simulink model "simulink_validacao"  (R2016a)
settings: Solver=VariableStepAuto  StartTime=0.0  StopTime=10.0  RelTol=1e-3
values from neighbouring files (symbols this model uses):
  f_mol_ar = [0.79 0.21 0.0 0 0 0 0 0]    [codigo_validacao.m]
  f_mol_gas = [0.76 0 0 0 0.11 0.13 0 0]    [codigo_validacao.m]
  m_c = 0.3    [codigo_validacao.m]
  m_f = 0.01    [codigo_validacao.m]
  N = 0.82    [codigo_validacao.m]
  Pc_i = 368000    [codigo_validacao.m]
  Ph_i = 105000    [codigo_validacao.m]
  Tc_i = 358.15    [codigo_validacao.m]
  Th_i = 584.817    [codigo_validacao.m]
(part 1 of 4)
settings Model: Creator=Janderson Honório  LastModifiedBy=Janderson Honório

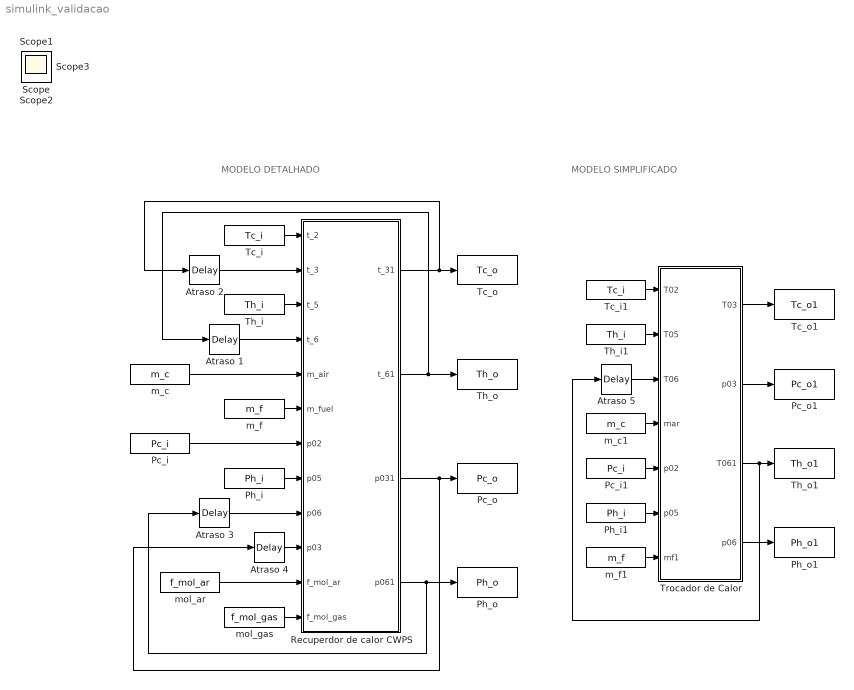
== system simulink_validacao ==
  note: MODELO DETALHADO
  note: MODELO SIMPLIFICADO
  Atraso 1 : TransportDelay  DelayTime=0.1  InitialOutput=400  TransDelayFeedthrough=on
  Atraso 2 : TransportDelay  DelayTime=0.1  InitialOutput=650  TransDelayFeedthrough=on
  Atraso 3 : TransportDelay  DelayTime=0.1  InitialOutput=300000  TransDelayFeedthrough=on
  Atraso 4 : TransportDelay  DelayTime=0.1  InitialOutput=100000  TransDelayFeedthrough=on
  Atraso 5 : TransportDelay  DelayTime=0.1  InitialOutput=500  TransDelayFeedthrough=on
  Pc_i : Constant  Value=Pc_i
  Pc_i1 : Constant  Value=Pc_i
  Pc_o : ToWorkspace  VariableName=Pc_o  SampleTime=-1
      settings: Save2DSignal=2-D array (concatenate along first dimension)
  Pc_o1 : ToWorkspace  VariableName=Pc_o1  SampleTime=-1
      settings: Save2DSignal=2-D array (concatenate along first dimension)
  Ph_i : Constant  Value=Ph_i
  Ph_i1 : Constant  Value=Ph_i
  Ph_o : ToWorkspace  VariableName=Ph_o  SampleTime=-1
      settings: Save2DSignal=2-D array (concatenate along first dimension)
  Ph_o1 : ToWorkspace  VariableName=Ph_o1  SampleTime=-1
      settings: Save2DSignal=2-D array (concatenate along first dimension)
  Recuperdor de calor CWPS : Subsystem
  Tc_i : Constant  Value=Tc_i
  Tc_i1 : Constant  Value=Tc_i
  Tc_o : ToWorkspace  VariableName=Tc_o  SampleTime=-1
      settings: Save2DSignal=2-D array (concatenate along first dimension)
  Tc_o1 : ToWorkspace  VariableName=Tc_o1  SampleTime=-1
      settings: Save2DSignal=2-D array (concatenate along first dimension)
  Th_i : Constant  Value=Th_i
  Th_i1 : Constant  Value=Th_i
  Th_o : ToWorkspace  VariableName=Th_o  SampleTime=-1
      settings: Save2DSignal=2-D array (concatenate along first dimension)
  Th_o1 : ToWorkspace  VariableName=Th_o1  SampleTime=-1
      settings: Save2DSignal=2-D array (concatenate along first dimension)
  Trocador de Calor : Subsystem
  m_c : Constant  Value=m_c
  m_c1 : Constant  Value=m_c
  m_f : Constant  Value=m_f
  m_f1 : Constant  Value=m_f
  mol_ar : Constant  Value=f_mol_ar
  mol_gas : Constant  Value=f_mol_gas
  Scope{,1..3} (4 alike) : Scope
  wires:
  Recuperdor de calor CWPS/1(t_31) -> Tc_o/1, Atraso 2/1
  Recuperdor de calor CWPS/2(t_61) -> Th_o/1, Atraso 1/1
  Recuperdor de calor CWPS/4(p061) -> Ph_o/1, Atraso 3/1
  Atraso 2/1 -> Recuperdor de calor CWPS/2(t_3)
  Th_i/1 -> Recuperdor de calor CWPS/3(t_5)
  Atraso 1/1 -> Recuperdor de calor CWPS/4(t_6)
  Atraso 4/1 -> Recuperdor de calor CWPS/10(p03)
  Atraso 3/1 -> Recuperdor de calor CWPS/9("p06 ")
  mol_ar/1 -> Recuperdor de calor CWPS/11(f_mol_ar)
  mol_gas/1 -> Recuperdor de calor CWPS/12(f_mol_gas)
  Tc_i/1 -> Recuperdor de calor CWPS/1(t_2)
  m_f/1 -> Recuperdor de calor CWPS/6(m_fuel)
  m_c/1 -> Recuperdor de calor CWPS/5("m_air ")
  Ph_i/1 -> Recuperdor de calor CWPS/8(p05)
  Pc_i/1 -> Recuperdor de calor CWPS/7(p02)
  Trocador de Calor/3(T061) -> Atraso 5/1, Th_o1/1
  Atraso 5/1 -> Trocador de Calor/3(T06)
  Tc_i1/1 -> Trocador de Calor/1(T02)
  Th_i1/1 -> Trocador de Calor/2(T05)
  m_c1/1 -> Trocador de Calor/4(mar)
  m_f1/1 -> Trocador de Calor/7(mf1)
  Pc_i1/1 -> Trocador de Calor/5(p02)
  Ph_i1/1 -> Trocador de Calor/6(p05)
  Trocador de Calor/1(T03) -> Tc_o1/1
  Trocador de Calor/2(p03) -> Pc_o1/1
  Trocador de Calor/4(p06) -> Ph_o1/1
  Recuperdor de calor CWPS/3(p031) -> Pc_o/1, Atraso 4/1

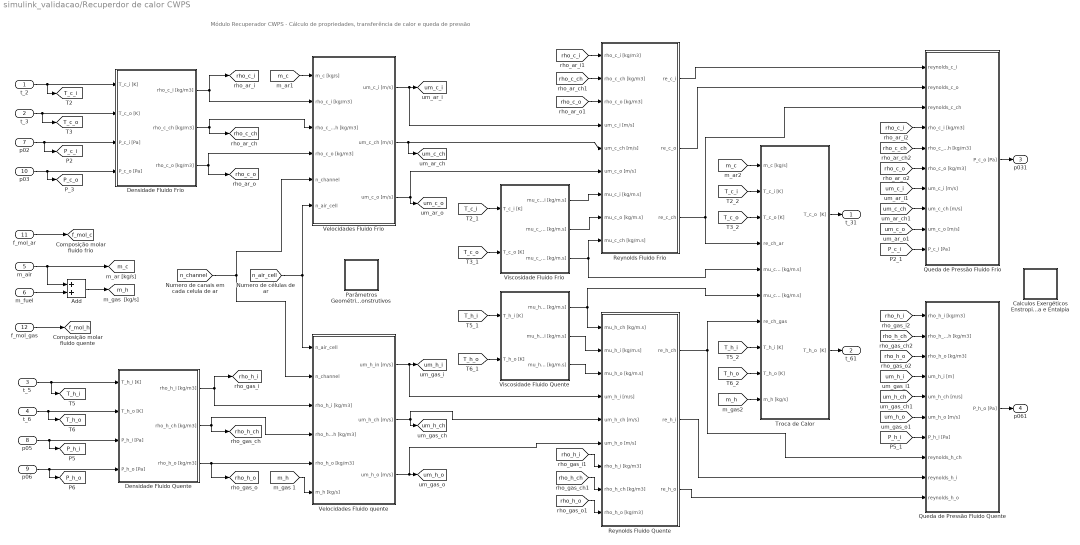
== system simulink_validacao/Recuperdor de calor CWPS ==
  note: Módulo Recuperador CWPS - Cálculo de propriedades, transferência de calor e queda de pressão
  t_2 : Inport
  t_3 : Inport  Port=2
  t_5 : Inport  Port=3
  t_6 : Inport  Port=4
  "m_air " : Inport  Port=5
  m_fuel : Inport  Port=6
  p02 : Inport  Port=7
  p05 : Inport  Port=8
  "p06 " : Inport  Port=9
  p03 : Inport  Port=10
  f_mol_ar : Inport  Port=11
  f_mol_gas : Inport  Port=12
  Add : Sum
  Calculos Exergéticos Enstropia e Entalpia : Subsystem
  Densidade Fluido Frio : Subsystem
  Densidade Fluido Quente : Subsystem
  Parâmetros Geométricos e Construtivos : Subsystem
  Queda de Pressão Fluido Frio : Subsystem
  Queda de Pressão Fluido Quente : Subsystem
  Reynolds Fluido Frio : Subsystem
  Reynolds Fluido Quente : Subsystem
  Troca de Calor : Subsystem
  Velocidades Fluido Frio : Subsystem
  Velocidades Fluido quente : Subsystem
  "Viscosidade Fluido Frio " : Subsystem
  Viscosidade Fluido Quente : Subsystem
  t_31 : Outport
  t_61 : Outport  Port=2
  p031 : Outport  Port=3
  p061 : Outport  Port=4
  tag scope: P_c_i=global, P_c_o=global, P_h_i=global, P_h_o=global, T_c_i=global, T_c_o=global, T_h_i=global, T_h_o=global, f_mol_c=global, f_mol_h=global, m_c=global, m_h=global, rho_c_ch=global, rho_c_i=global, rho_c_o=global, rho_h_ch=global, rho_h_i=global, rho_h_o=global, um_c_ch=global, um_c_i=global, um_c_o=global, um_h_ch=global, um_h_i=global, um_h_o=global
  wires:
  t_3/1 -> [T_c_o], Densidade Fluido Frio/2(T_c_o [K])
  t_2/1 -> Densidade Fluido Frio/1(T_c_i [K]), [T_c_i]
  p02/1 -> [P_c_i], Densidade Fluido Frio/3(P_c_i [Pa])
  t_6/1 -> [T_h_o], Densidade Fluido Quente/2(T_h_o [K])
  t_5/1 -> [T_h_i], Densidade Fluido Quente/1(T_h_i [K])
  "p06 "/1 -> [P_h_o], Densidade Fluido Quente/4(P_h_o [Pa])
  Densidade Fluido Frio/2(rho_c_ch [kg/m3]) -> Velocidades Fluido Frio/3(rho_c_ch [kg/m3]), [rho_c_ch]
  Densidade Fluido Frio/3(rho_c_o [kg/m3]) -> [rho_c_o], Velocidades Fluido Frio/4("rho_c_o [kg/m3] ")
  Densidade Fluido Quente/2(rho_h_ch [kg/m3]) -> Velocidades Fluido quente/4(rho_h_ch [kg/m3]), [rho_h_ch]
  Densidade Fluido Quente/3(rho_h_o [kg/m3]) -> Velocidades Fluido quente/5(rho_h_o [kg/m3]), [rho_h_o]
  Densidade Fluido Quente/1(rho_h_i [kg/m3]) -> [rho_h_i], Velocidades Fluido quente/3(rho_h_i [kg/m3])
  [n_air_cell] -> Velocidades Fluido quente/1(n_air_cell), Velocidades Fluido Frio/6(n_air_cell)
  [n_channel] -> Velocidades Fluido quente/2(n_channel), Velocidades Fluido Frio/5(n_channel)
  Velocidades Fluido Frio/1(um_c_i [m/s]) -> [um_c_i], Reynolds Fluido Frio/4(um_c_i [m/s])
  Velocidades Fluido Frio/2(um_c_ch [m/s]) -> [um_c_ch], Reynolds Fluido Frio/5(um_c_ch [m/s])
  Velocidades Fluido Frio/3(um_c_o [m/s]) -> Reynolds Fluido Frio/6(um_c_o [m/s]), [um_c_o]
  Velocidades Fluido quente/1(um_h_in [m/s]) -> [um_h_i], Reynolds Fluido Quente/4(um_h_i [m/s])
  Velocidades Fluido quente/2(um_h_ch [m/s]) -> Reynolds Fluido Quente/5(um_h_ch [m/s]), [um_h_ch]
  Velocidades Fluido quente/3(um_h_o [m/s]) -> Reynolds Fluido Quente/6(um_h_o [m/s]), [um_h_o]
  Queda de Pressão Fluido Quente/1(P_h_o [Pa]) -> p061/1
  p05/1 -> [P_h_i], Densidade Fluido Quente/3(P_h_i [Pa])
  [rho_c_i] -> Reynolds Fluido Frio/1(rho_c_i [kg/m3])
  [rho_c_ch] -> Reynolds Fluido Frio/2(rho_c_ch [kg/m3])
  [rho_c_o] -> Reynolds Fluido Frio/3(rho_c_o [kg/m3])
  [rho_c_i] -> Queda de Pressão Fluido Frio/4(rho_c_i [kg/m3])
  [rho_c_o] -> Queda de Pressão Fluido Frio/6("rho_c_o [kg/m3] ")
  [rho_c_ch] -> Queda de Pressão Fluido Frio/5("rho_c_ch [kg/m3] ")
  [rho_h_i] -> Reynolds Fluido Quente/7(rho_h_i [kg/m3])
  [rho_h_ch] -> Reynolds Fluido Quente/8(rho_h_ch [kg/m3])
  [rho_h_o] -> Reynolds Fluido Quente/9(rho_h_o [kg/m3])
  [rho_h_o] -> Queda de Pressão Fluido Quente/3("rho_h_o [kg/m3] ")
  [rho_h_i] -> Queda de Pressão Fluido Quente/1(rho_h_i [kg/m3])
  [rho_h_ch] -> Queda de Pressão Fluido Quente/2("rho_h_ch [kg/m3] ")
  Troca de Calor/2(T_h_o  [K]) -> t_61/1
  [um_c_i] -> Queda de Pressão Fluido Frio/7(um_c_i [m/s])
  [um_c_ch] -> Queda de Pressão Fluido Frio/8(um_c_ch [m/s])
  [um_c_o] -> Queda de Pressão Fluido Frio/9(um_c_o [m/s])
  [um_h_i] -> Queda de Pressão Fluido Quente/4(um_h_i [m])
  [um_h_ch] -> Queda de Pressão Fluido Quente/5(um_h_ch [m/s])
  [um_h_o] -> Queda de Pressão Fluido Quente/6(um_h_o [m/s])
  [T_c_i] -> "Viscosidade Fluido Frio "/1(T_c_i [K])
  [T_c_o] -> "Viscosidade Fluido Frio "/2(T_c_o [K])
  [P_h_i] -> Queda de Pressão Fluido Quente/7(P_h_i [Pa])
  [P_c_i] -> Queda de Pressão Fluido Frio/10(P_c_i [Pa])
  "m_air "/1 -> Add/1, [m_c]
  [m_c] -> Velocidades Fluido Frio/1(m_c [kg/s])
  [m_h] -> Velocidades Fluido quente/6(m_h [kg/s])
  [m_h] -> Troca de Calor/10(m_h [kg/s])
  Troca de Calor/1(T_c_o  [K]) -> t_31/1
  [m_c] -> Troca de Calor/1(m_c [kg/s])
  [T_h_i] -> Troca de Calor/8(T_h_i [K])
  [T_h_o] -> Troca de Calor/9(T_h_o [K])
  [T_c_i] -> Troca de Calor/2("T_c_i [K] ")
  [T_c_o] -> Troca de Calor/3(T_c_o [K])
  [T_h_i] -> Viscosidade Fluido Quente/1(T_h_i [K])
  [T_h_o] -> Viscosidade Fluido Quente/2(T_h_o [K])
  "Viscosidade Fluido Frio "/2(mu_c_o [kg/m.s]) -> Reynolds Fluido Frio/8(mu_c_o [kg/m.s])
  "Viscosidade Fluido Frio "/3(mu_c_ch [kg/m.s]) -> Troca de Calor/5(mu_ch_c [kg/m.s]), Reynolds Fluido Frio/9(mu_c_ch [kg/m.s])
  "Viscosidade Fluido Frio "/1(mu_c_i [kg/m.s]) -> Reynolds Fluido Frio/7(mu_c_i [kg/m.s])
  Viscosidade Fluido Quente/1(mu_h_ch [kg/m.s]) -> Troca de Calor/6(mu_ch_h [kg/m.s]), Reynolds Fluido Quente/1(mu_h_ch [kg/m.s])
  Viscosidade Fluido Quente/2(mu_h_i [kg/m.s]) -> Reynolds Fluido Quente/2("mu_h_i [kg/m.s] ")
  Viscosidade Fluido Quente/3(mu_h_o [kg/m.s]) -> Reynolds Fluido Quente/3(mu_h_o [kg/m.s])
  Reynolds Fluido Frio/3(re_c_ch) -> Troca de Calor/4(re_ch_ar), Queda de Pressão Fluido Frio/3(reynolds_c_ch)
  Reynolds Fluido Quente/1(re_h_ch) -> Troca de Calor/7(re_ch_gas), Queda de Pressão Fluido Quente/8(reynolds_h_ch)
  Reynolds Fluido Frio/1(re_c_i) -> Queda de Pressão Fluido Frio/1(reynolds_c_i)
  Reynolds Fluido Frio/2(re_c_o) -> Queda de Pressão Fluido Frio/2(reynolds_c_o)
  Reynolds Fluido Quente/2(re_h_i) -> Queda de Pressão Fluido Quente/9(reynolds_h_i)
  Reynolds Fluido Quente/3(re_h_o) -> Queda de Pressão Fluido Quente/10(reynolds_h_o)
  p03/1 -> [P_c_o], Densidade Fluido Frio/4(P_c_o [Pa])
  Densidade Fluido Frio/1(rho_c_i [kg/m3]) -> Velocidades Fluido Frio/2(rho_c_i [kg/m3]), [rho_c_i]
  f_mol_ar/1 -> [f_mol_c]
  f_mol_gas/1 -> [f_mol_h]
  Queda de Pressão Fluido Frio/1(P_c_o [Pa]) -> p031/1
  m_fuel/1 -> Add/2
  Add/1 -> [m_h]

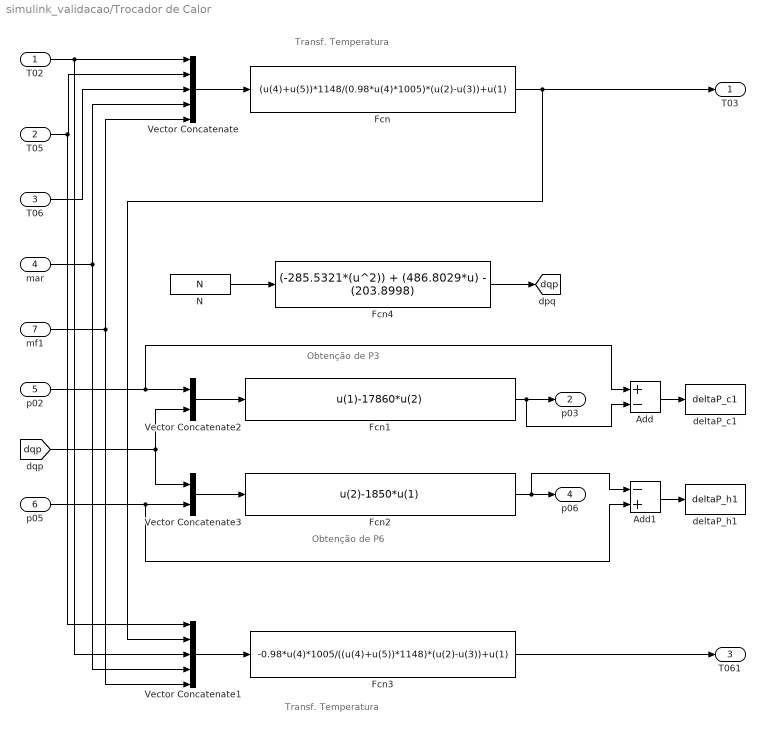
== system simulink_validacao/Trocador de Calor ==
  note: Transf. Temperatura
  note: Obtenção de P3
  note: Obtenção de P6
  note: Transf. Temperatura
  T02 : Inport
  T05 : Inport  Port=2
  T06 : Inport  Port=3
  mar : Inport  Port=4
  p02 : Inport  Port=5
  p05 : Inport  Port=6
  mf1 : Inport  Port=7
  Add : Sum  Inputs=+-
  Add1 : Sum  Inputs=-+
  Fcn : Fcn  Expr=(u(4)+u(5))*1148/(0.98*u(4)*1005)*(u(2)-u(3))+u(1)
  Fcn1 : Fcn  Expr=u(1)-17860*u(2)
  Fcn2 : Fcn  Expr=u(2)-1850*u(1)
  Fcn3 : Fcn  Expr=-0.98*u(4)*1005/((u(4)+u(5))*1148)*(u(2)-u(3))+u(1)
  Fcn4 : Fcn  Expr=(-285.5321*(u^2)) + (486.8029*u) - (203.8998)
  N : Constant  Value=N
  Vector Concatenate : Concatenate  NumInputs=5
  Vector Concatenate1 : Concatenate  NumInputs=5
  Vector Concatenate2 : Concatenate
  Vector Concatenate3 : Concatenate
  deltaP_c1 : ToWorkspace  VariableName=deltaP_c1  SampleTime=-1
      settings: Save2DSignal=2-D array (concatenate along first dimension)
  deltaP_h1 : ToWorkspace  VariableName=deltaP_h1  SampleTime=-1
      settings: Save2DSignal=2-D array (concatenate along first dimension)
  T03 : Outport
  p03 : Outport  Port=2
  T061 : Outport  Port=3
  p06 : Outport  Port=4
  tag scope: dqp=global
  wires:
  Fcn3/1 -> T061/1
  Vector Concatenate/1 -> Fcn/1
  Fcn1/1 -> Add/2, p03/1
  T06/1 -> Vector Concatenate/3
  Fcn2/1 -> Add1/1, p06/1
  Vector Concatenate1/1 -> Fcn3/1
  T05/1 -> Vector Concatenate1/1, Vector Concatenate/2
  Fcn/1 -> Vector Concatenate1/2, T03/1
  T02/1 -> Vector Concatenate1/3, Vector Concatenate/1
  mar/1 -> Vector Concatenate1/4, Vector Concatenate/4
  mf1/1 -> Vector Concatenate1/5, Vector Concatenate/5
  p02/1 -> Add/1, Vector Concatenate2/1
  [dqp] -> Vector Concatenate3/1, Vector Concatenate2/2
  Vector Concatenate2/1 -> Fcn1/1
  p05/1 -> Add1/2, Vector Concatenate3/2
  Vector Concatenate3/1 -> Fcn2/1
  N/1 -> Fcn4/1
  Fcn4/1 -> [dqp]
  Add1/1 -> deltaP_h1/1
  Add/1 -> deltaP_c1/1

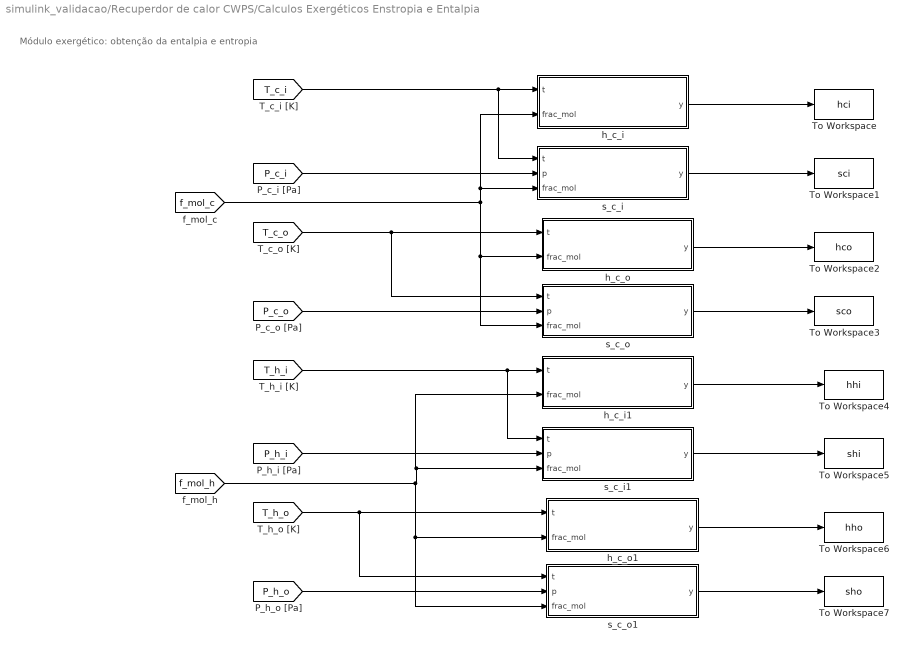
== system simulink_validacao/Recuperdor de calor CWPS/Calculos Exergéticos Enstropia e Entalpia ==
  note: Módulo exergético: obtenção da entalpia e entropia
  To Workspace : ToWorkspace  VariableName=hci  SampleTime=-1
      settings: Save2DSignal=2-D array (concatenate along first dimension)
  To Workspace1 : ToWorkspace  VariableName=sci  SampleTime=-1
      settings: Save2DSignal=2-D array (concatenate along first dimension)
  To Workspace2 : ToWorkspace  VariableName=hco  SampleTime=-1
      settings: Save2DSignal=2-D array (concatenate along first dimension)
  To Workspace3 : ToWorkspace  VariableName=sco  SampleTime=-1
      settings: Save2DSignal=2-D array (concatenate along first dimension)
  To Workspace4 : ToWorkspace  VariableName=hhi  SampleTime=-1
      settings: Save2DSignal=2-D array (concatenate along first dimension)
  To Workspace5 : ToWorkspace  VariableName=shi  SampleTime=-1
      settings: Save2DSignal=2-D array (concatenate along first dimension)
  To Workspace6 : ToWorkspace  VariableName=hho  SampleTime=-1
      settings: Save2DSignal=2-D array (concatenate along first dimension)
  To Workspace7 : ToWorkspace  VariableName=sho  SampleTime=-1
      settings: Save2DSignal=2-D array (concatenate along first dimension)
  h_c_i : MATLAB Function  TreatAsAtomicUnit=on
  h_c_i1 : MATLAB Function  TreatAsAtomicUnit=on
  h_c_o : MATLAB Function  TreatAsAtomicUnit=on
  h_c_o1 : MATLAB Function  TreatAsAtomicUnit=on
  s_c_i : MATLAB Function  TreatAsAtomicUnit=on
  s_c_i1 : MATLAB Function  TreatAsAtomicUnit=on
  s_c_o : MATLAB Function  TreatAsAtomicUnit=on
  s_c_o1 : MATLAB Function  TreatAsAtomicUnit=on
  wires:
  [T_c_i] -> s_c_i/1(t), h_c_i/1(t)
  [f_mol_c] -> s_c_o/3(frac_mol), h_c_o/2(frac_mol), h_c_i/2(frac_mol), s_c_i/3(frac_mol)
  h_c_i/1(y) -> To Workspace/1
  s_c_i/1(y) -> To Workspace1/1
  [P_c_i] -> s_c_i/2(p)
  h_c_o/1(y) -> To Workspace2/1
  s_c_o/1(y) -> To Workspace3/1
  h_c_i1/1(y) -> To Workspace4/1
  s_c_i1/1(y) -> To Workspace5/1
  h_c_o1/1(y) -> To Workspace6/1
  s_c_o1/1(y) -> To Workspace7/1
  [T_c_o] -> h_c_o/1(t), s_c_o/1(t)
  [P_c_o] -> s_c_o/2(p)
  [T_h_i] -> s_c_i1/1(t), h_c_i1/1(t)
  [P_h_i] -> s_c_i1/2(p)
  [f_mol_h] -> s_c_o1/3(frac_mol), h_c_o1/2(frac_mol), s_c_i1/3(frac_mol), h_c_i1/2(frac_mol)
  [T_h_o] -> s_c_o1/1(t), h_c_o1/1(t)
  [P_h_o] -> s_c_o1/2(p)

== system simulink_validacao/Recuperdor de calor CWPS/Densidade Fluido Frio ==
  note: Módulo cálculo de densidades no recuperador - Fluido frio
  T_c_i [K] : Inport
  T_c_o [K] : Inport  Port=2
  P_c_i [Pa] : Inport  Port=3
  P_c_o [Pa] : Inport  Port=4
  Mux : Mux  Inputs=2
  Mux2 : Mux  Inputs=2
  P media fluido frio : Fcn  Expr=(u(1)+u(2))/2
  T media fluido frio : Fcn  Expr=(u(1)+u(2))/2
  densidade_c_ch : MATLAB Function  TreatAsAtomicUnit=on
  densidade_c_i : MATLAB Function  TreatAsAtomicUnit=on
  densidade_c_o : MATLAB Function  TreatAsAtomicUnit=on
  rho_c_i [kg/m3] : Outport
  rho_c_ch [kg/m3] : Outport  Port=2
  rho_c_o [kg/m3] : Outport  Port=3
  wires:
  Mux/1 -> T media fluido frio/1
  T_c_i [K]/1 -> densidade_c_i/1(t), Mux/1
  densidade_c_ch/1(y) -> rho_c_ch [kg/m3]/1
  densidade_c_i/1(y) -> rho_c_i [kg/m3]/1
  densidade_c_o/1(y) -> rho_c_o [kg/m3]/1
  Mux2/1 -> P media fluido frio/1
  T media fluido frio/1 -> densidade_c_ch/1(t)
  P media fluido frio/1 -> densidade_c_ch/2(p)
  T_c_o [K]/1 -> densidade_c_o/1(t), Mux/2
  P_c_i [Pa]/1 -> Mux2/1, densidade_c_i/2(p)
  P_c_o [Pa]/1 -> densidade_c_o/2(p), Mux2/2
  [f_mol_c] -> densidade_c_o/3(frac_mol), densidade_c_ch/3(frac_mol), densidade_c_i/3(frac_mol)

== system simulink_validacao/Recuperdor de calor CWPS/Densidade Fluido Quente ==
  note: Módulo cálculo de densidades no recuperador - Fluido quente
  T_h_i [K] : Inport
  T_h_o [K] : Inport  Port=2
  P_h_i [Pa] : Inport  Port=3
  P_h_o [Pa] : Inport  Port=4
  Mux1 : Mux  Inputs=2
  Mux3 : Mux  Inputs=2
  P media fluido quente : Fcn  Expr=(u(1)+u(2))/2
  T media fluido quente : Fcn  Expr=(u(1)+u(2))/2
  densidade_h_ch : MATLAB Function  TreatAsAtomicUnit=on
  densidade_h_i : MATLAB Function  TreatAsAtomicUnit=on
  densidade_h_o : MATLAB Function  TreatAsAtomicUnit=on
  rho_h_i [kg/m3] : Outport
  rho_h_ch [kg/m3] : Outport  Port=2
  rho_h_o [kg/m3] : Outport  Port=3
  wires:
  Mux1/1 -> T media fluido quente/1
  T_h_i [K]/1 -> Mux1/1, densidade_h_i/1(t)
  Mux3/1 -> P media fluido quente/1
  T media fluido quente/1 -> densidade_h_ch/1(t)
  P media fluido quente/1 -> densidade_h_ch/2(p)
  T_h_o [K]/1 -> densidade_h_o/1(t), Mux1/2
  P_h_i [Pa]/1 -> densidade_h_i/2(p), Mux3/1
  P_h_o [Pa]/1 -> densidade_h_o/2(p), Mux3/2
  densidade_h_i/1(y) -> rho_h_i [kg/m3]/1
  densidade_h_ch/1(y) -> rho_h_ch [kg/m3]/1
  densidade_h_o/1(y) -> rho_h_o [kg/m3]/1
  [f_mol_h] -> densidade_h_i/3(frac_mol), densidade_h_o/3(frac_mol), densidade_h_ch/3(frac_mol)

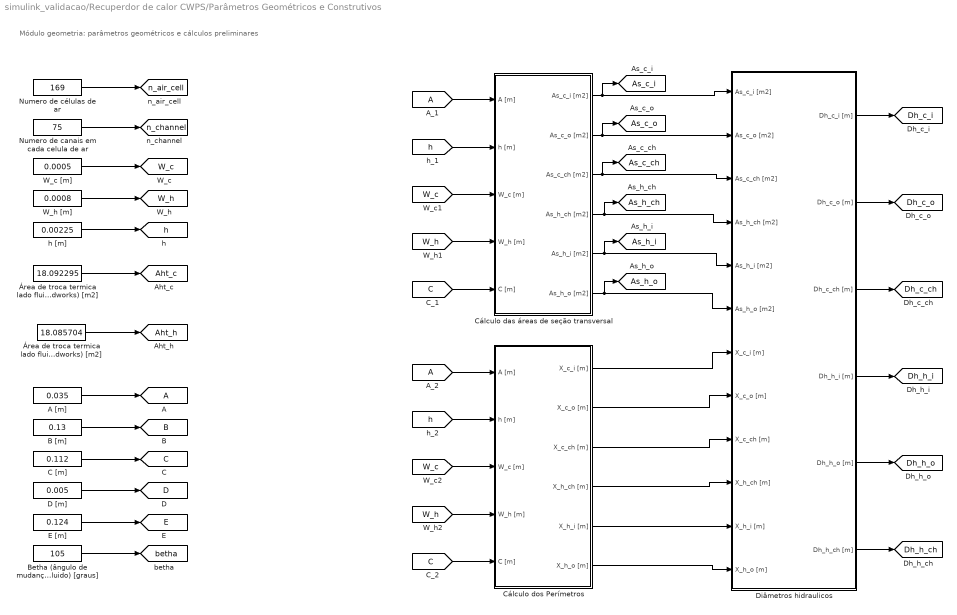
== system simulink_validacao/Recuperdor de calor CWPS/Parâmetros Geométricos e Construtivos ==
  note: Módulo geometria: parâmetros geométricos e cálculos preliminares
  A [m] : Constant  Value=0.035
  B [m] : Constant  Value=0.13
  Betha (ângulo de mudança de direção do fluido) [graus] : Constant  Value=105
  C [m] : Constant  Value=0.112
  Cálculo das áreas de seção transversal : Subsystem
  Cálculo dos Perímetros : Subsystem
  D [m] : Constant  Value=0.005
  "Diâmetros hidraulicos " : Subsystem
  E [m] : Constant  Value=0.124
  Numero de canais em cada celula de ar : Constant  Value=75
  Numero de células de ar : Constant  Value=169
  W_c [m] : Constant  Value=0.0005
  W_h [m] : Constant  Value=0.0008
  h [m] : Constant  Value=0.00225
  Área de troca termica lado fluido frio (Obtido via Solidworks) [m2] : Constant  Value=18.092295
  Área de troca termica lado fluido quente (Obtido via Solidworks) [m2] : Constant  Value=18.085704
  tag scope: A=global, Aht_c=global, Aht_h=global, As_c_ch=global, As_c_i=global, As_c_o=global, As_h_ch=global, As_h_i=global, As_h_o=global, B=global, C=global, D=global, Dh_c_ch=global, Dh_c_i=global, Dh_c_o=global, Dh_h_ch=global, Dh_h_i=global, Dh_h_o=global, E=global, W_c=global, W_h=global, betha=global, h=global, n_air_cell=global, n_channel=global
  wires:
  Numero de células de ar/1 -> [n_air_cell]
  Numero de canais em cada celula de ar/1 -> [n_channel]
  W_c [m]/1 -> [W_c]
  W_h [m]/1 -> [W_h]
  h [m]/1 -> [h]
  E [m]/1 -> [E]
  D [m]/1 -> [D]
  C [m]/1 -> [C]
  B [m]/1 -> [B]
  A [m]/1 -> [A]
  Betha (ângulo de mudança de direção do fluido) [graus]/1 -> [betha]
  [A] -> Cálculo das áreas de seção transversal/1(A [m])
  [h] -> Cálculo das áreas de seção transversal/2(h [m])
  [W_c] -> Cálculo das áreas de seção transversal/3(W_c [m])
  [W_h] -> Cálculo das áreas de seção transversal/4(W_h [m])
  [C] -> Cálculo das áreas de seção transversal/5(C [m])
  [A] -> Cálculo dos Perímetros/1(A [m])
  [h] -> Cálculo dos Perímetros/2(h [m])
  [W_c] -> Cálculo dos Perímetros/3(W_c [m])
  [W_h] -> Cálculo dos Perímetros/4(W_h [m])
  [C] -> Cálculo dos Perímetros/5(C [m])
  "Diâmetros hidraulicos "/1(Dh_c_i [m]) -> [Dh_c_i]
  "Diâmetros hidraulicos "/3(Dh_c_ch [m]) -> [Dh_c_ch]
  "Diâmetros hidraulicos "/4(Dh_h_i [m]) -> [Dh_h_i]
  "Diâmetros hidraulicos "/5(Dh_h_o [m]) -> [Dh_h_o]
  "Diâmetros hidraulicos "/6(Dh_h_ch [m]) -> [Dh_h_ch]
  Cálculo das áreas de seção transversal/1(As_c_i [m2]) -> [As_c_i], "Diâmetros hidraulicos "/1(As_c_i [m2])
  Cálculo das áreas de seção transversal/2(As_c_o [m2]) -> [As_c_o], "Diâmetros hidraulicos "/2(As_c_o [m2])
  Cálculo das áreas de seção transversal/3(As_c_ch [m2]) -> [As_c_ch], "Diâmetros hidraulicos "/3(As_c_ch [m2])
  Cálculo das áreas de seção transversal/4(As_h_ch [m2]) -> [As_h_ch], "Diâmetros hidraulicos "/4(As_h_ch [m2])
  Cálculo das áreas de seção transversal/5(As_h_i [m2]) -> [As_h_i], "Diâmetros hidraulicos "/5(As_h_i [m2])
  Cálculo das áreas de seção transversal/6(As_h_o [m2]) -> [As_h_o], "Diâmetros hidraulicos "/6(As_h_o [m2])
  Cálculo dos Perímetros/1(X_c_i [m]) -> "Diâmetros hidraulicos "/7(X_c_i [m])
  Cálculo dos Perímetros/2(X_c_o [m]) -> "Diâmetros hidraulicos "/8(X_c_o [m])
  Cálculo dos Perímetros/3(X_c_ch [m]) -> "Diâmetros hidraulicos "/9(X_c_ch [m])
  Cálculo dos Perímetros/4(X_h_ch [m]) -> "Diâmetros hidraulicos "/10(X_h_ch [m])
  Cálculo dos Perímetros/5(X_h_i [m]) -> "Diâmetros hidraulicos "/11(X_h_i [m])
  Cálculo dos Perímetros/6(X_h_o [m]) -> "Diâmetros hidraulicos "/12(X_h_o [m])
  "Diâmetros hidraulicos "/2(Dh_c_o [m]) -> [Dh_c_o]
  Área de troca termica lado fluido frio (Obtido via Solidworks) [m2]/1 -> [Aht_c]
  Área de troca termica lado fluido quente (Obtido via Solidworks) [m2]/1 -> [Aht_h]

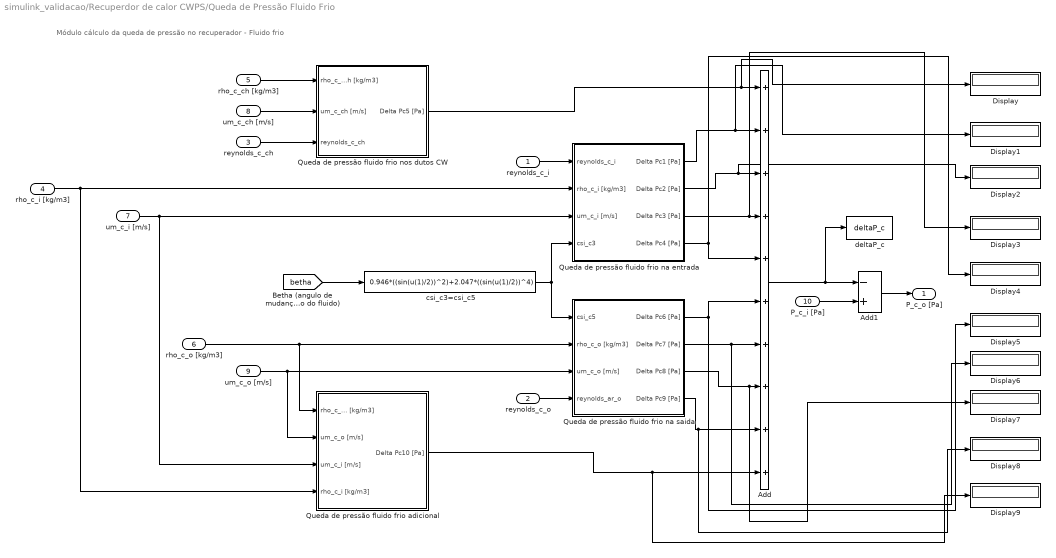
== system simulink_validacao/Recuperdor de calor CWPS/Queda de Pressão Fluido Frio ==
  note: Módulo cálculo da queda de pressão no recuperador - Fluido frio
  reynolds_c_i : Inport
  reynolds_c_o : Inport  Port=2
  reynolds_c_ch : Inport  Port=3
  rho_c_i [kg/m3] : Inport  Port=4
  "rho_c_ch [kg/m3] " : Inport  Port=5
  "rho_c_o [kg/m3] " : Inport  Port=6
  um_c_i [m/s] : Inport  Port=7
  um_c_ch [m/s] : Inport  Port=8
  um_c_o [m/s] : Inport  Port=9
  P_c_i [Pa] : Inport  Port=10
  Add : Sum  Inputs=10
  Add1 : Sum  Inputs=-+
  Display{,1..9} (10 alike) : Display
  "Queda de pressão fluido frio adicional " : Subsystem
  Queda de pressão fluido frio na entrada : Subsystem
  Queda de pressão fluido frio nos dutos CW : Subsystem
  "Queda de pressão fluido frio na saida " : Subsystem
  csi_c3=csi_c5 : Fcn  Expr=0.946*((sin(u(1)/2))^2)+2.047*((sin(u(1)/2))^4)
  deltaP_c : ToWorkspace  VariableName=deltaP_c  SampleTime=-1
      settings: Save2DSignal=2-D array (concatenate along first dimension)
  P_c_o [Pa] : Outport
  wires:
  [betha] -> csi_c3=csi_c5/1
  reynolds_c_o/1 -> "Queda de pressão fluido frio na saida "/4(reynolds_ar_o)
  reynolds_c_ch/1 -> Queda de pressão fluido frio nos dutos CW/3(reynolds_c_ch)
  "rho_c_ch [kg/m3] "/1 -> Queda de pressão fluido frio nos dutos CW/1(rho_c_ch [kg/m3])
  um_c_ch [m/s]/1 -> Queda de pressão fluido frio nos dutos CW/2(um_c_ch [m/s])
  csi_c3=csi_c5/1 -> Queda de pressão fluido frio na entrada/4(csi_c3), "Queda de pressão fluido frio na saida "/1(csi_c5)
  reynolds_c_i/1 -> Queda de pressão fluido frio na entrada/1(reynolds_c_i)
  rho_c_i [kg/m3]/1 -> Queda de pressão fluido frio na entrada/2(rho_c_i [kg/m3]), "Queda de pressão fluido frio adicional "/4(rho_c_i [kg/m3])
  um_c_i [m/s]/1 -> Queda de pressão fluido frio na entrada/3(um_c_i [m/s]), "Queda de pressão fluido frio adicional "/3(um_c_i [m/s])
  um_c_o [m/s]/1 -> "Queda de pressão fluido frio adicional "/2(um_c_o [m/s]), "Queda de pressão fluido frio na saida "/3(um_c_o [m/s])
  "rho_c_o [kg/m3] "/1 -> "Queda de pressão fluido frio adicional "/1(rho_c_o [kg/m3]), "Queda de pressão fluido frio na saida "/2(rho_c_o [kg/m3])
  Queda de pressão fluido frio nos dutos CW/1(Delta Pc5 [Pa]) -> Display/1, Add/1
  Queda de pressão fluido frio na entrada/1(Delta Pc1 [Pa]) -> Display1/1, Add/2
  Queda de pressão fluido frio na entrada/2(Delta Pc2 [Pa]) -> Display2/1, Add/3
  Queda de pressão fluido frio na entrada/3(Delta Pc3 [Pa]) -> Display3/1, Add/4
  Queda de pressão fluido frio na entrada/4(Delta Pc4 [Pa]) -> Display4/1, Add/5
  "Queda de pressão fluido frio na saida "/1(Delta Pc6 [Pa]) -> Add/6, Display5/1
  "Queda de pressão fluido frio na saida "/2(Delta Pc7 [Pa]) -> Display6/1, Add/7
  "Queda de pressão fluido frio na saida "/3(Delta Pc8 [Pa]) -> Display7/1, Add/8
  "Queda de pressão fluido frio na saida "/4(Delta Pc9 [Pa]) -> Display8/1, Add/9
  "Queda de pressão fluido frio adicional "/1(Delta Pc10 [Pa]) -> Display9/1, Add/10
  Add/1 -> deltaP_c/1, Add1/1
  P_c_i [Pa]/1 -> Add1/2
  Add1/1 -> P_c_o [Pa]/1

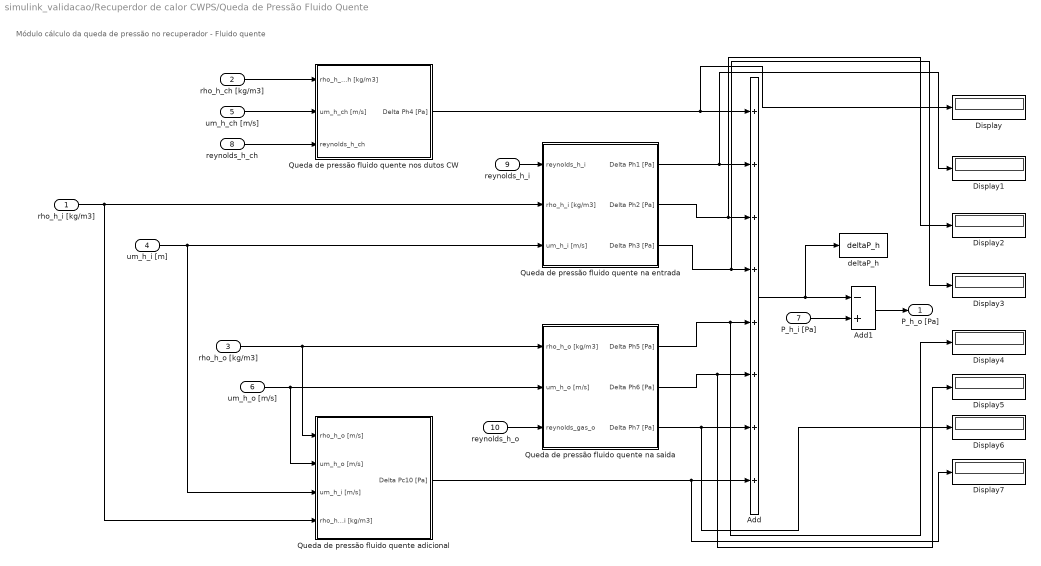
== system simulink_validacao/Recuperdor de calor CWPS/Queda de Pressão Fluido Quente ==
  note: Módulo cálculo da queda de pressão no recuperador - Fluido quente
  rho_h_i [kg/m3] : Inport
  "rho_h_ch [kg/m3] " : Inport  Port=2
  "rho_h_o [kg/m3] " : Inport  Port=3
  um_h_i [m] : Inport  Port=4
  um_h_ch [m/s] : Inport  Port=5
  um_h_o [m/s] : Inport  Port=6
  P_h_i [Pa] : Inport  Port=7
  reynolds_h_ch : Inport  Port=8
  reynolds_h_i : Inport  Port=9
  reynolds_h_o : Inport  Port=10
  Add : Sum  Inputs=8
  Add1 : Sum  Inputs=-+
  Display{,1..7} (8 alike) : Display
  Queda de pressão fluido quente na saida : Subsystem
  "Queda de pressão fluido quente adicional " : Subsystem
  Queda de pressão fluido quente na entrada : Subsystem
  Queda de pressão fluido quente nos dutos CW : Subsystem
  deltaP_h : ToWorkspace  VariableName=deltaP_h  SampleTime=-1
      settings: Save2DSignal=2-D array (concatenate along first dimension)
  P_h_o [Pa] : Outport
  wires:
  reynolds_h_ch/1 -> Queda de pressão fluido quente nos dutos CW/3(reynolds_h_ch)
  "rho_h_ch [kg/m3] "/1 -> Queda de pressão fluido quente nos dutos CW/1(rho_h_ch [kg/m3])
  um_h_ch [m/s]/1 -> Queda de pressão fluido quente nos dutos CW/2(um_h_ch [m/s])
  reynolds_h_i/1 -> Queda de pressão fluido quente na entrada/1(reynolds_h_i)
  rho_h_i [kg/m3]/1 -> "Queda de pressão fluido quente adicional "/4(rho_h_i [kg/m3]), Queda de pressão fluido quente na entrada/2(rho_h_i [kg/m3])
  um_h_i [m]/1 -> "Queda de pressão fluido quente adicional "/3(um_h_i [m/s]), Queda de pressão fluido quente na entrada/3(um_h_i [m/s])
  um_h_o [m/s]/1 -> Queda de pressão fluido quente na saida/2(um_h_o [m/s]), "Queda de pressão fluido quente adicional "/2(um_h_o [m/s])
  Queda de pressão fluido quente nos dutos CW/1(Delta Ph4 [Pa]) -> Display/1, Add/1
  Queda de pressão fluido quente na entrada/1(Delta Ph1 [Pa]) -> Display1/1, Add/2
  Queda de pressão fluido quente na entrada/2(Delta Ph2 [Pa]) -> Display2/1, Add/3
  Queda de pressão fluido quente na entrada/3(Delta Ph3 [Pa]) -> Display3/1, Add/4
  "Queda de pressão fluido quente adicional "/1(Delta Pc10 [Pa]) -> Display7/1, Add/8
  "rho_h_o [kg/m3] "/1 -> "Queda de pressão fluido quente adicional "/1(rho_h_o [m/s]), Queda de pressão fluido quente na saida/1(rho_h_o [kg/m3])
  reynolds_h_o/1 -> Queda de pressão fluido quente na saida/3(reynolds_gas_o)
  Queda de pressão fluido quente na saida/3(Delta Ph7 [Pa]) -> Display6/1, Add/7
  Queda de pressão fluido quente na saida/2(Delta Ph6 [Pa]) -> Display5/1, Add/6
  Queda de pressão fluido quente na saida/1(Delta Ph5 [Pa]) -> Display4/1, Add/5
  Add/1 -> deltaP_h/1, Add1/1
  P_h_i [Pa]/1 -> Add1/2
  Add1/1 -> P_h_o [Pa]/1

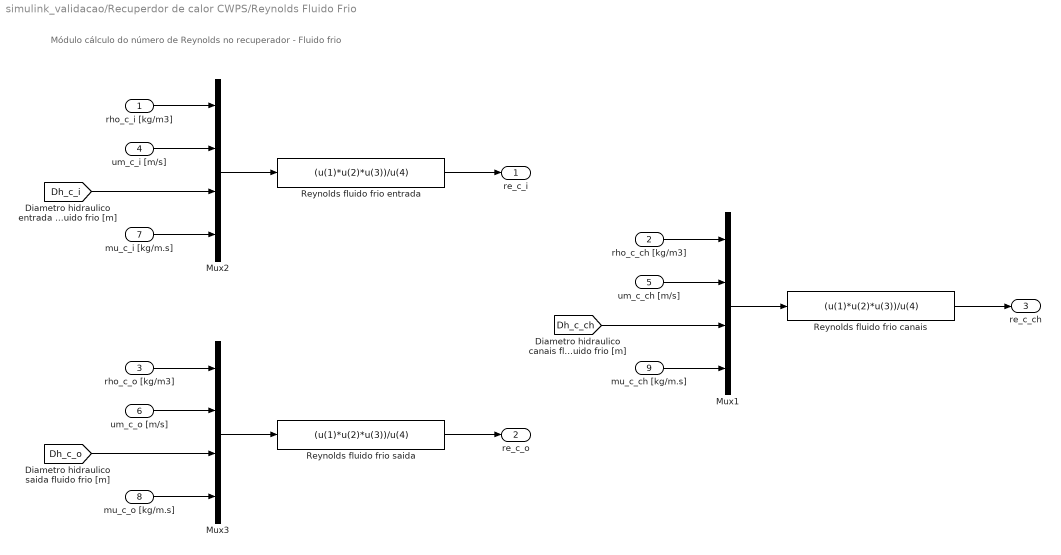
== system simulink_validacao/Recuperdor de calor CWPS/Reynolds Fluido Frio ==
  note: Módulo cálculo do número de Reynolds no recuperador - Fluido frio
  rho_c_i [kg/m3] : Inport
  rho_c_ch [kg/m3] : Inport  Port=2
  rho_c_o [kg/m3] : Inport  Port=3
  um_c_i [m/s] : Inport  Port=4
  um_c_ch [m/s] : Inport  Port=5
  um_c_o [m/s] : Inport  Port=6
  mu_c_i [kg/m.s] : Inport  Port=7
  mu_c_o [kg/m.s] : Inport  Port=8
  mu_c_ch [kg/m.s] : Inport  Port=9
  Mux1 : Mux
  Mux2 : Mux
  Mux3 : Mux
  Reynolds fluido frio canais : Fcn  Expr=(u(1)*u(2)*u(3))/u(4)
  Reynolds fluido frio entrada : Fcn  Expr=(u(1)*u(2)*u(3))/u(4)
  Reynolds fluido frio saida : Fcn  Expr=(u(1)*u(2)*u(3))/u(4)
  re_c_i : Outport
  re_c_o : Outport  Port=2
  re_c_ch : Outport  Port=3
  wires:
  Reynolds fluido frio entrada/1 -> re_c_i/1
  Mux2/1 -> Reynolds fluido frio entrada/1
  [Dh_c_i] -> Mux2/3
  mu_c_i [kg/m.s]/1 -> Mux2/4
  um_c_i [m/s]/1 -> Mux2/2
  Reynolds fluido frio canais/1 -> re_c_ch/1
  Mux1/1 -> Reynolds fluido frio canais/1
  [Dh_c_ch] -> Mux1/3
  mu_c_ch [kg/m.s]/1 -> Mux1/4
  um_c_ch [m/s]/1 -> Mux1/2
  rho_c_ch [kg/m3]/1 -> Mux1/1
  Reynolds fluido frio saida/1 -> re_c_o/1
  Mux3/1 -> Reynolds fluido frio saida/1
  [Dh_c_o] -> Mux3/3
  mu_c_o [kg/m.s]/1 -> Mux3/4
  um_c_o [m/s]/1 -> Mux3/2
  rho_c_o [kg/m3]/1 -> Mux3/1
  rho_c_i [kg/m3]/1 -> Mux2/1

== system simulink_validacao/Recuperdor de calor CWPS/Reynolds Fluido Quente ==
  note: Módulo cálculo do número de Reynolds no recuperador - Fluido quente
  mu_h_ch [kg/m.s] : Inport
  "mu_h_i [kg/m.s] " : Inport  Port=2
  mu_h_o [kg/m.s] : Inport  Port=3
  um_h_i [m/s] : Inport  Port=4
  um_h_ch [m/s] : Inport  Port=5
  um_h_o [m/s] : Inport  Port=6
  rho_h_i [kg/m3] : Inport  Port=7
  rho_h_ch [kg/m3] : Inport  Port=8
  rho_h_o [kg/m3] : Inport  Port=9
  Mux1 : Mux
  Mux2 : Mux
  Mux3 : Mux
  Reynolds fluido quente canais : Fcn  Expr=(u(1)*u(2)*u(3))/u(4)
  Reynolds fluido quente entrada : Fcn  Expr=(u(1)*u(2)*u(3))/u(4)
  Reynolds fluido quente saida : Fcn  Expr=(u(1)*u(2)*u(3))/u(4)
  re_h_ch : Outport
  re_h_i : Outport  Port=2
  re_h_o : Outport  Port=3
  wires:
  Reynolds fluido quente entrada/1 -> re_h_i/1
  Mux2/1 -> Reynolds fluido quente entrada/1
  [Dh_h_i] -> Mux2/3
  "mu_h_i [kg/m.s] "/1 -> Mux2/4
  um_h_i [m/s]/1 -> Mux2/2
  Reynolds fluido quente canais/1 -> re_h_ch/1
  Mux1/1 -> Reynolds fluido quente canais/1
  mu_h_ch [kg/m.s]/1 -> Mux1/4
  um_h_ch [m/s]/1 -> Mux1/2
  rho_h_ch [kg/m3]/1 -> Mux1/1
  Reynolds fluido quente saida/1 -> re_h_o/1
  Mux3/1 -> Reynolds fluido quente saida/1
  [Dh_h_o] -> Mux3/3
  mu_h_o [kg/m.s]/1 -> Mux3/4
  um_h_o [m/s]/1 -> Mux3/2
  rho_h_o [kg/m3]/1 -> Mux3/1
  rho_h_i [kg/m3]/1 -> Mux2/1
  [Dh_h_ch] -> Mux1/3

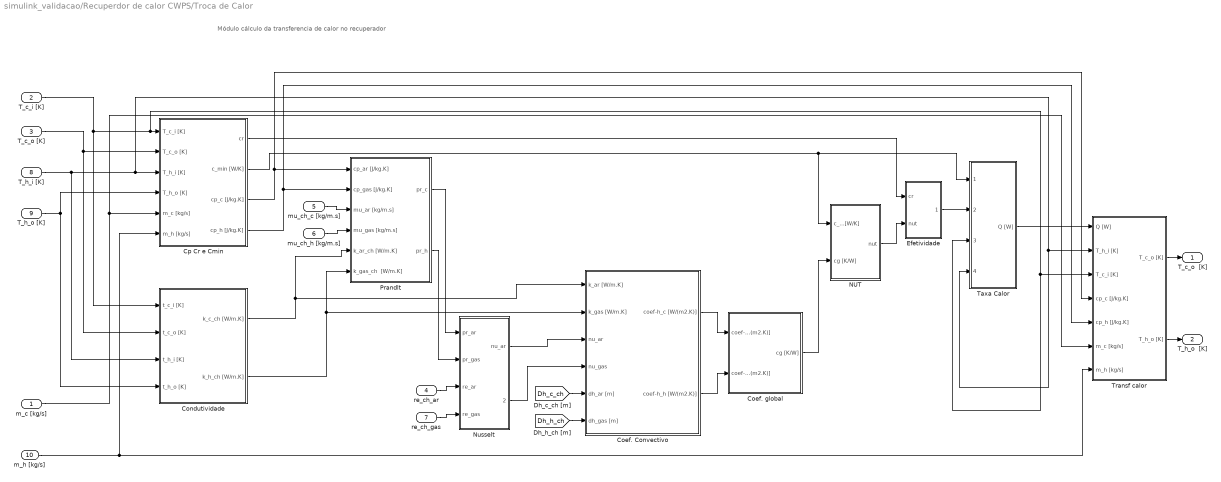
== system simulink_validacao/Recuperdor de calor CWPS/Troca de Calor ==
  note: Módulo cálculo da transferencia de calor no recuperador
  m_c [kg/s] : Inport
  "T_c_i [K] " : Inport  Port=2
  T_c_o [K] : Inport  Port=3
  re_ch_ar : Inport  Port=4
  mu_ch_c [kg/m.s] : Inport  Port=5
  mu_ch_h [kg/m.s] : Inport  Port=6
  re_ch_gas : Inport  Port=7
  T_h_i [K] : Inport  Port=8
  T_h_o [K] : Inport  Port=9
  m_h [kg/s] : Inport  Port=10
  Coef. Convectivo : Subsystem
  Coef. global : Subsystem
  Condutividade : Subsystem
  Cp Cr e Cmin : Subsystem
  Efetividade : Subsystem
  NUT : Subsystem
  Nusselt : Subsystem
  Prandlt : Subsystem
  Taxa Calor : Subsystem
  Transf calor : Subsystem
  T_c_o  [K] : Outport
  T_h_o  [K] : Outport  Port=2
  wires:
  Transf calor/1(T_c_o [K]) -> T_c_o  [K]/1
  Cp Cr e Cmin/4(cp_h [J/kg.K]) -> Transf calor/5(cp_h [J/kg.K]), Prandlt/2(cp_gas [J/kg.K])
  Condutividade/2(k_h_ch [W/m.K]) -> Prandlt/6(k_gas_ch  [W/m.K]), Coef. Convectivo/2(k_gas [W/m.K])
  Efetividade/1(epsilon) -> Taxa Calor/2(epsilon)
  Prandlt/2(pr_h) -> Nusselt/2(pr_gas)
  Coef. global/1(cg [K/W]) -> NUT/2(cg [K/W])
  re_ch_ar/1 -> Nusselt/3(re_ar)
  Coef. Convectivo/2(coef-h_h [W/(m2.K)]) -> Coef. global/2(coef-h_h [W/(m2.K)])
  NUT/1(nut) -> Efetividade/2(nut)
  Coef. Convectivo/1(coef-h_c [W/(m2.K)]) -> Coef. global/1(coef-h_c [W/(m2.K)])
  Nusselt/1(nu_ar) -> Coef. Convectivo/3(nu_ar)
  Prandlt/1(pr_c) -> Nusselt/1(pr_ar)
  Cp Cr e Cmin/2(c_min [W/K]) -> Taxa Calor/1(c_min [W/K]), NUT/1(c_min [W/K])
  Taxa Calor/1(Q [W]) -> Transf calor/1(Q [W])
  Nusselt/2(nu_gas) -> Coef. Convectivo/4(nu_gas)
  Cp Cr e Cmin/3(cp_c [J/kg.K]) -> Transf calor/4(cp_c [J/kg.K]), Prandlt/1(cp_ar [J/kg.K])
  re_ch_gas/1 -> Nusselt/4(re_gas)
  Transf calor/2(T_h_o [K]) -> T_h_o  [K]/1
  Condutividade/1(k_c_ch [W/m.K]) -> Prandlt/5(k_ar_ch [W/m.K]), Coef. Convectivo/1(k_ar [W/m.K])
  Cp Cr e Cmin/1(cr) -> Efetividade/1(cr)
  T_h_o [K]/1 -> Condutividade/4(t_h_o [K]), Cp Cr e Cmin/4(T_h_o [K])
  m_c [kg/s]/1 -> Transf calor/6(m_c [kg/s]), Cp Cr e Cmin/5(m_c [kg/s])
  m_h [kg/s]/1 -> Cp Cr e Cmin/6(m_h [kg/s]), Transf calor/7("m_h [kg/s] ")
  "T_c_i [K] "/1 -> Condutividade/1(t_c_i [K]), Taxa Calor/3(T_c_i [K]), Transf calor/3(T_c_i [K]), Cp Cr e Cmin/1(T_c_i [K])
  T_c_o [K]/1 -> Condutividade/2(t_c_o [K]), Cp Cr e Cmin/2(T_c_o [K])
  T_h_i [K]/1 -> Condutividade/3(t_h_i [K]), Cp Cr e Cmin/3(T_h_i [K]), Taxa Calor/4(T_h_i [K]), Transf calor/2(T_h_i [K])
  mu_ch_c [kg/m.s]/1 -> Prandlt/3(mu_ar [kg/m.s])
  mu_ch_h [kg/m.s]/1 -> Prandlt/4(mu_gas [kg/m.s])
  [Dh_c_ch] -> Coef. Convectivo/5(dh_ar [m])
  [Dh_h_ch] -> Coef. Convectivo/6(dh_gas [m])

== system simulink_validacao/Recuperdor de calor CWPS/Velocidades Fluido Frio ==
  note: Módulo cálculo de velocidade média no recuperador - Fluido frio
  m_c [kg/s] : Inport
  rho_c_i [kg/m3] : Inport  Port=2
  rho_c_ch [kg/m3] : Inport  Port=3
  "rho_c_o [kg/m3] " : Inport  Port=4
  n_channel : Inport  Port=5
  n_air_cell : Inport  Port=6
  Mux1 : Mux  Inputs=3
  Mux2 : Mux  Inputs=3
  Mux3 : Mux  Inputs=3
  Velocidade fluido frio canais : Fcn  Expr=u(1)/(u(2)*u(3))
  Velocidade fluido frio entrada : Fcn  Expr=u(1)/(u(2)*u(3))
  Velocidade fluido frio saida : Fcn  Expr=u(1)/(u(2)*u(3))
  vazão/(n_canais*n_aircel) : Product  Inputs=*//
  vazão/n_aircel : Product  Inputs=*/
  um_c_i [m/s] : Outport
  um_c_ch [m/s] : Outport  Port=2
  um_c_o [m/s] : Outport  Port=3
  wires:
  Velocidade fluido frio entrada/1 -> um_c_i [m/s]/1
  Mux2/1 -> Velocidade fluido frio entrada/1
  rho_c_i [kg/m3]/1 -> Mux2/3
  Velocidade fluido frio canais/1 -> um_c_ch [m/s]/1
  Mux1/1 -> Velocidade fluido frio canais/1
  [As_c_ch] -> Mux1/2
  rho_c_ch [kg/m3]/1 -> Mux1/3
  Velocidade fluido frio saida/1 -> um_c_o [m/s]/1
  Mux3/1 -> Velocidade fluido frio saida/1
  [As_c_o] -> Mux3/2
  "rho_c_o [kg/m3] "/1 -> Mux3/3
  m_c [kg/s]/1 -> vazão/n_aircel/1, vazão/(n_canais*n_aircel)/1
  vazão/(n_canais*n_aircel)/1 -> Mux1/1
  n_channel/1 -> vazão/(n_canais*n_aircel)/3
  n_air_cell/1 -> vazão/n_aircel/2, vazão/(n_canais*n_aircel)/2
  vazão/n_aircel/1 -> Mux2/1, Mux3/1
  [As_c_i] -> Mux2/2

== system simulink_validacao/Recuperdor de calor CWPS/Velocidades Fluido quente ==
  note: Módulo cálculo de velocidade média no recuperador - Fluido quente
  n_air_cell : Inport
  n_channel : Inport  Port=2
  rho_h_i [kg/m3] : Inport  Port=3
  rho_h_ch [kg/m3] : Inport  Port=4
  rho_h_o [kg/m3] : Inport  Port=5
  m_h [kg/s] : Inport  Port=6
  Mux1 : Mux  Inputs=3
  Mux2 : Mux  Inputs=3
  Mux3 : Mux  Inputs=3
  Velocidade fluido quente canais : Fcn  Expr=u(1)/(u(2)*u(3))
  Velocidade fluido quente entrada : Fcn  Expr=u(1)/(u(2)*u(3))
  Velocidade fluido quente saida : Fcn  Expr=u(1)/(u(2)*u(3))
  vazão/(n_canais*n_aircel) : Product  Inputs=*//
  vazão/n_aircel : Product  Inputs=*/
  um_h_in [m/s] : Outport
  um_h_ch [m/s] : Outport  Port=2
  um_h_o [m/s] : Outport  Port=3
  wires:
  Velocidade fluido quente entrada/1 -> um_h_in [m/s]/1
  Mux2/1 -> Velocidade fluido quente entrada/1
  rho_h_i [kg/m3]/1 -> Mux2/3
  Velocidade fluido quente canais/1 -> um_h_ch [m/s]/1
  Mux1/1 -> Velocidade fluido quente canais/1
  rho_h_ch [kg/m3]/1 -> Mux1/3
  Velocidade fluido quente saida/1 -> um_h_o [m/s]/1
  Mux3/1 -> Velocidade fluido quente saida/1
  rho_h_o [kg/m3]/1 -> Mux3/3
  vazão/(n_canais*n_aircel)/1 -> Mux1/1
  n_channel/1 -> vazão/(n_canais*n_aircel)/3
  n_air_cell/1 -> vazão/n_aircel/2, vazão/(n_canais*n_aircel)/2
  vazão/n_aircel/1 -> Mux2/1, Mux3/1
  m_h [kg/s]/1 -> vazão/n_aircel/1, vazão/(n_canais*n_aircel)/1
  [As_h_ch] -> Mux1/2
  [As_h_o] -> Mux3/2
  [As_h_i] -> Mux2/2

== system simulink_validacao/Recuperdor de calor CWPS/Viscosidade Fluido Frio  ==
  note: Módulo cálculo de viscosidades no recuperador - Fluido frio
  T_c_i [K] : Inport
  T_c_o [K] : Inport  Port=2
  Mux : Mux  Inputs=2
  T media fluido frio : Fcn  Expr=(u(1)+u(2))/2
  visc_c_c : MATLAB Function  TreatAsAtomicUnit=on
  visc_c_ch : MATLAB Function  TreatAsAtomicUnit=on
  visc_c_o : MATLAB Function  TreatAsAtomicUnit=on
  mu_c_i [kg/m.s] : Outport
  mu_c_o [kg/m.s] : Outport  Port=2
  mu_c_ch [kg/m.s] : Outport  Port=3
  wires:
  Mux/1 -> T media fluido frio/1
  T_c_i [K]/1 -> visc_c_c/1(t), Mux/1
  T_c_o [K]/1 -> visc_c_o/1(t), Mux/2
  T media fluido frio/1 -> visc_c_ch/1(t)
  visc_c_ch/1(y) -> mu_c_ch [kg/m.s]/1
  visc_c_c/1(y) -> mu_c_i [kg/m.s]/1
  visc_c_o/1(y) -> mu_c_o [kg/m.s]/1
  [f_mol_c] -> visc_c_c/2(frac_mol), visc_c_o/2(frac_mol), visc_c_ch/2(frac_mol)

== system simulink_validacao/Recuperdor de calor CWPS/Viscosidade Fluido Quente ==
  note: Módulo cálculo de viscosidades no recuperador - Fluido quente
  T_h_i [K] : Inport
  T_h_o [K] : Inport  Port=2
  Mux1 : Mux  Inputs=2
  T media fluido quente : Fcn  Expr=(u(1)+u(2))/2
  visc_h_ch : MATLAB Function  TreatAsAtomicUnit=on
  visc_h_i : MATLAB Function  TreatAsAtomicUnit=on
  visc_h_o : MATLAB Function  TreatAsAtomicUnit=on
  mu_h_ch [kg/m.s] : Outport
  mu_h_i [kg/m.s] : Outport  Port=2
  mu_h_o [kg/m.s] : Outport  Port=3
  wires:
  Mux1/1 -> T media fluido quente/1
  T_h_i [K]/1 -> visc_h_i/1(t), Mux1/1
  T_h_o [K]/1 -> visc_h_o/1(t), Mux1/2
  T media fluido quente/1 -> visc_h_ch/1(t)
  visc_h_ch/1(y) -> mu_h_ch [kg/m.s]/1
  visc_h_i/1(y) -> mu_h_i [kg/m.s]/1
  visc_h_o/1(y) -> mu_h_o [kg/m.s]/1
  [f_mol_h] -> visc_h_o/2(frac_mol), visc_h_ch/2(frac_mol), visc_h_i/2(frac_mol)

== system simulink_validacao/Recuperdor de calor CWPS/Parâmetros Geométricos e Construtivos/Cálculo das áreas de seção transversal ==
  A [m] : Inport
  h [m] : Inport  Port=2
  W_c [m] : Inport  Port=3
  W_h [m] : Inport  Port=4
  C [m] : Inport  Port=5
  "Area seção transversal fluido frio entrada/saida " : Fcn  Expr=u(1)*2*u(2)
  Area seção transversal fluido frio nos canais : Fcn  Expr=u(1)*2*u(2)+((-4+pi)/4)*(u(2)^2-u(3)^2)
  Area seção transversal fluido quente entrada/saida : Fcn  Expr=u(1)*2*u(2)
  Area seção transversal fluido quente nos canais : Fcn  Expr=u(1)*2*u(3)+((-4+pi)/4)*(u(3)^2-u(2)^2)
  Mux1 : Mux  Inputs=2
  Mux2 : Mux  Inputs=2
  Mux3 : Mux  Inputs=3
  As_c_i [m2] : Outport
  As_c_o [m2] : Outport  Port=2
  As_c_ch [m2] : Outport  Port=3
  As_h_ch [m2] : Outport  Port=4
  As_h_i [m2] : Outport  Port=5
  As_h_o [m2] : Outport  Port=6
  wires:
  Mux2/1 -> "Area seção transversal fluido frio entrada/saida "/1
  Area seção transversal fluido quente entrada/saida/1 -> As_h_i [m2]/1, As_h_o [m2]/1
  C [m]/1 -> Mux1/1
  h [m]/1 -> Mux1/2, Mux3/1, Mux2/2
  Mux1/1 -> Area seção transversal fluido quente entrada/saida/1
  "Area seção transversal fluido frio entrada/saida "/1 -> As_c_o [m2]/1, As_c_i [m2]/1
  A [m]/1 -> Mux2/1
  W_h [m]/1 -> Mux3/3
  Mux3/1 -> Area seção transversal fluido frio nos canais/1, Area seção transversal fluido quente nos canais/1
  W_c [m]/1 -> Mux3/2
  Area seção transversal fluido frio nos canais/1 -> As_c_ch [m2]/1
  Area seção transversal fluido quente nos canais/1 -> As_h_ch [m2]/1

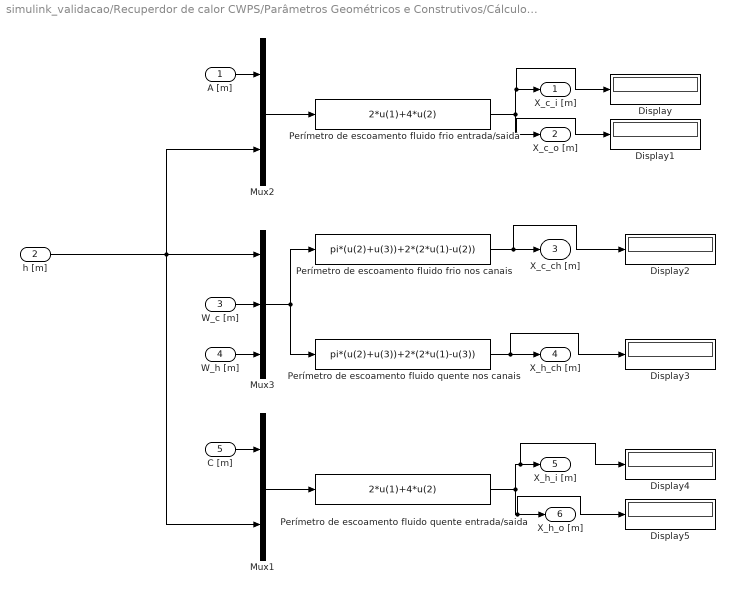
== system simulink_validacao/Recuperdor de calor CWPS/Parâmetros Geométricos e Construtivos/Cálculo dos Perímetros ==
  A [m] : Inport
  h [m] : Inport  Port=2
  W_c [m] : Inport  Port=3
  W_h [m] : Inport  Port=4
  C [m] : Inport  Port=5
  Display{,1..5} (6 alike) : Display
  Mux1 : Mux  Inputs=2
  Mux2 : Mux  Inputs=2
  Mux3 : Mux  Inputs=3
  "Perímetro de escoamento fluido frio entrada/saida " : Fcn  Expr=2*u(1)+4*u(2)
  Perímetro de escoamento fluido frio nos canais : Fcn  Expr=pi*(u(2)+u(3))+2*(2*u(1)-u(2))
  Perímetro de escoamento fluido quente entrada/saida : Fcn  Expr=2*u(1)+4*u(2)
  Perímetro de escoamento fluido quente nos canais : Fcn  Expr=pi*(u(2)+u(3))+2*(2*u(1)-u(3))
  X_c_i [m] : Outport
  X_c_o [m] : Outport  Port=2
  X_c_ch [m] : Outport  Port=3
  X_h_ch [m] : Outport  Port=4
  X_h_i [m] : Outport  Port=5
  X_h_o [m] : Outport  Port=6
  wires:
  Mux2/1 -> "Perímetro de escoamento fluido frio entrada/saida "/1
  Perímetro de escoamento fluido quente entrada/saida/1 -> Display4/1, X_h_i [m]/1, Display5/1, X_h_o [m]/1
  C [m]/1 -> Mux1/1
  h [m]/1 -> Mux1/2, Mux3/1, Mux2/2
  Mux1/1 -> Perímetro de escoamento fluido quente entrada/saida/1
  "Perímetro de escoamento fluido frio entrada/saida "/1 -> Display1/1, X_c_o [m]/1, Display/1, X_c_i [m]/1
  A [m]/1 -> Mux2/1
  W_h [m]/1 -> Mux3/3
  Mux3/1 -> Perímetro de escoamento fluido frio nos canais/1, Perímetro de escoamento fluido quente nos canais/1
  W_c [m]/1 -> Mux3/2
  Perímetro de escoamento fluido frio nos canais/1 -> Display2/1, X_c_ch [m]/1
  Perímetro de escoamento fluido quente nos canais/1 -> Display3/1, X_h_ch [m]/1

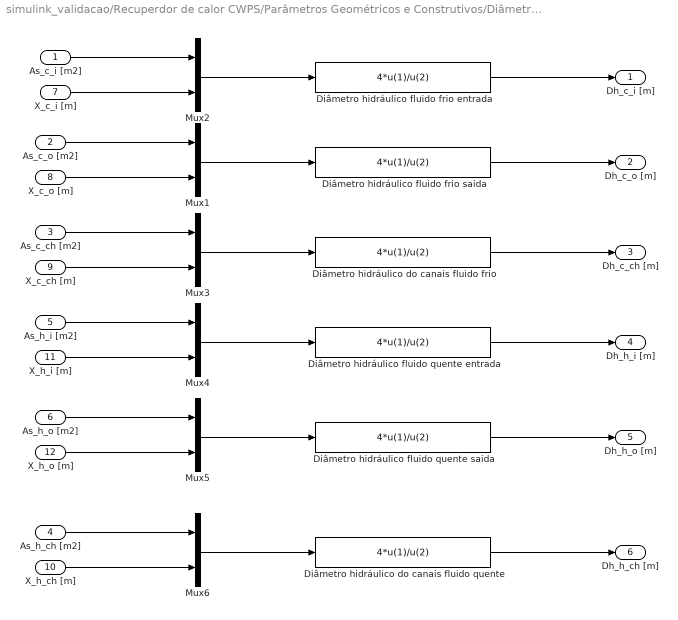
== system simulink_validacao/Recuperdor de calor CWPS/Parâmetros Geométricos e Construtivos/Diâmetros hidraulicos  ==
  As_c_i [m2] : Inport
  As_c_o [m2] : Inport  Port=2
  As_c_ch [m2] : Inport  Port=3
  As_h_ch [m2] : Inport  Port=4
  As_h_i [m2] : Inport  Port=5
  As_h_o [m2] : Inport  Port=6
  X_c_i [m] : Inport  Port=7
  X_c_o [m] : Inport  Port=8
  X_c_ch [m] : Inport  Port=9
  X_h_ch [m] : Inport  Port=10
  X_h_i [m] : Inport  Port=11
  X_h_o [m] : Inport  Port=12
  "Diâmetro hidráulico do canais fluido frio " : Fcn  Expr=4*u(1)/u(2)
  Diâmetro hidráulico do canais fluido quente : Fcn  Expr=4*u(1)/u(2)
  Diâmetro hidráulico fluido frio entrada : Fcn  Expr=4*u(1)/u(2)
  Diâmetro hidráulico fluido frio saida : Fcn  Expr=4*u(1)/u(2)
  Diâmetro hidráulico fluido quente entrada : Fcn  Expr=4*u(1)/u(2)
  Diâmetro hidráulico fluido quente saida : Fcn  Expr=4*u(1)/u(2)
  Mux{1..6} (6 alike) : Mux  Inputs=2
  Dh_c_i [m] : Outport
  Dh_c_o [m] : Outport  Port=2
  Dh_c_ch [m] : Outport  Port=3
  Dh_h_i [m] : Outport  Port=4
  Dh_h_o [m] : Outport  Port=5
  Dh_h_ch [m] : Outport  Port=6
  wires:
  Mux6/1 -> Diâmetro hidráulico do canais fluido quente/1
  Diâmetro hidráulico do canais fluido quente/1 -> Dh_h_ch [m]/1
  Mux5/1 -> Diâmetro hidráulico fluido quente saida/1
  Diâmetro hidráulico fluido quente saida/1 -> Dh_h_o [m]/1
  Diâmetro hidráulico fluido frio saida/1 -> Dh_c_o [m]/1
  Mux1/1 -> Diâmetro hidráulico fluido frio saida/1
  Mux4/1 -> Diâmetro hidráulico fluido quente entrada/1
  Diâmetro hidráulico fluido quente entrada/1 -> Dh_h_i [m]/1
  Diâmetro hidráulico fluido frio entrada/1 -> Dh_c_i [m]/1
  Mux3/1 -> "Diâmetro hidráulico do canais fluido frio "/1
  "Diâmetro hidráulico do canais fluido frio "/1 -> Dh_c_ch [m]/1
  Mux2/1 -> Diâmetro hidráulico fluido frio entrada/1
  As_c_i [m2]/1 -> Mux2/1
  As_c_ch [m2]/1 -> Mux3/1
  As_h_i [m2]/1 -> Mux4/1
  As_h_o [m2]/1 -> Mux5/1
  As_h_ch [m2]/1 -> Mux6/1
  X_c_i [m]/1 -> Mux2/2
  X_c_o [m]/1 -> Mux1/2
  X_c_ch [m]/1 -> Mux3/2
  X_h_i [m]/1 -> Mux4/2
  X_h_o [m]/1 -> Mux5/2
  X_h_ch [m]/1 -> Mux6/2
  As_c_o [m2]/1 -> Mux1/1

== system simulink_validacao/Recuperdor de calor CWPS/Queda de Pressão Fluido Frio/Queda de pressão fluido frio adicional  ==
  rho_c_o [kg/m3] : Inport
  um_c_o [m/s] : Inport  Port=2
  um_c_i [m/s] : Inport  Port=3
  rho_c_i [kg/m3] : Inport  Port=4
  Delta P c10 : Fcn  Expr=(u(1)*u(2)^2)-(u(3)*u(4)^2)
  Mux9 : Mux
  Delta Pc10 [Pa] : Outport
  wires:
  Delta P c10/1 -> Delta Pc10 [Pa]/1
  Mux9/1 -> Delta P c10/1
  rho_c_o [kg/m3]/1 -> Mux9/1
  um_c_o [m/s]/1 -> Mux9/2
  rho_c_i [kg/m3]/1 -> Mux9/3
  um_c_i [m/s]/1 -> Mux9/4

== system simulink_validacao/Recuperdor de calor CWPS/Queda de Pressão Fluido Frio/Queda de pressão fluido frio na entrada ==
  reynolds_c_i : Inport
  rho_c_i [kg/m3] : Inport  Port=2
  um_c_i [m/s] : Inport  Port=3
  csi_c3 : Inport  Port=4
  Delta P c1 : Fcn  Expr=u(3)*((u(1)*u(2)^2)/2)
  Delta P c2 : Fcn  Expr=u(3)*(u(4)/(2*u(5)))*((u(1)*u(2)^2)/2)
  Delta P c3 : Fcn  Expr=u(3)*((u(1)*u(2)^2)/2)
  Delta P c4 : Fcn  Expr=u(3)*((u(1)*u(2)^2)/2)
  Fator de atrito fluido frio entrada : Fcn  Expr=112/u(1)
  Mux2 : Mux  Inputs=3
  Mux3 : Mux  Inputs=5
  Mux4 : Mux  Inputs=3
  csi_c1=csi_c2 : Constant  Value=0.5
  Delta Pc1 [Pa] : Outport
  Delta Pc2 [Pa] : Outport  Port=2
  Delta Pc3 [Pa] : Outport  Port=3
  Delta Pc4 [Pa] : Outport  Port=4
  wires:
  Mux2/1 -> Delta P c1/1, Delta P c3/1
  Delta P c4/1 -> Delta Pc4 [Pa]/1
  [E] -> Mux3/4
  csi_c1=csi_c2/1 -> Mux2/3
  Mux3/1 -> Delta P c2/1
  [Dh_c_i] -> Mux3/5
  Mux4/1 -> Delta P c4/1
  Fator de atrito fluido frio entrada/1 -> Mux3/3
  Delta P c1/1 -> Delta Pc1 [Pa]/1
  um_c_i [m/s]/1 -> Mux4/2, Mux2/2, Mux3/2
  reynolds_c_i/1 -> Fator de atrito fluido frio entrada/1
  Delta P c2/1 -> Delta Pc2 [Pa]/1
  Delta P c3/1 -> Delta Pc3 [Pa]/1
  csi_c3/1 -> Mux4/3
  rho_c_i [kg/m3]/1 -> Mux3/1, Mux4/1, Mux2/1

== system simulink_validacao/Recuperdor de calor CWPS/Queda de Pressão Fluido Frio/Queda de pressão fluido frio nos dutos CW ==
  rho_c_ch [kg/m3] : Inport
  um_c_ch [m/s] : Inport  Port=2
  reynolds_c_ch : Inport  Port=3
  Delta P c5 : Fcn  Expr=u(3)*(u(4)/u(5))*((u(1)*u(2)^2)/2)
  Display : Display
  Fator de atrito fluido frio canais : Fcn  Expr=u(2)*(112/u(1))
  Mux1 : Mux  Inputs=2
  Mux8 : Mux  Inputs=5
  kappa : Constant  Value=1.6
  Delta Pc5 [Pa] : Outport
  wires:
  Mux8/1 -> Delta P c5/1
  um_c_ch [m/s]/1 -> Mux8/2
  rho_c_ch [kg/m3]/1 -> Mux8/1
  [Dh_c_ch] -> Mux8/5
  Fator de atrito fluido frio canais/1 -> Mux8/3
  Delta P c5/1 -> Delta Pc5 [Pa]/1
  Mux1/1 -> Fator de atrito fluido frio canais/1
  reynolds_c_ch/1 -> Display/1, Mux1/1
  kappa/1 -> Mux1/2
  [B] -> Mux8/4

== system simulink_validacao/Recuperdor de calor CWPS/Queda de Pressão Fluido Frio/Queda de pressão fluido frio na saida  ==
  csi_c5 : Inport
  rho_c_o [kg/m3] : Inport  Port=2
  um_c_o [m/s] : Inport  Port=3
  reynolds_ar_o : Inport  Port=4
  Delta P c6 : Fcn  Expr=u(3)*((u(1)*u(2)^2)/2)
  Delta P c7 : Fcn  Expr=u(3)*((u(1)*u(2)^2)/2)
  Delta P c8 : Fcn  Expr=u(3)*(u(4)/(2*u(5)))*((u(1)*u(2)^2)/2)
  Delta P c9 : Fcn  Expr=u(3)*((u(1)*u(2)^2)/2)
  Fator de atrito saída : Fcn  Expr=112/u(1)
  Mux5 : Mux  Inputs=3
  Mux6 : Mux  Inputs=3
  Mux7 : Mux  Inputs=5
  csi_c4=csi_c6 : Constant
  Delta Pc6 [Pa] : Outport
  Delta Pc7 [Pa] : Outport  Port=2
  Delta Pc8 [Pa] : Outport  Port=3
  Delta Pc9 [Pa] : Outport  Port=4
  wires:
  Fator de atrito saída/1 -> Mux7/3
  rho_c_o [kg/m3]/1 -> Mux7/1, Mux5/1, Mux6/1
  um_c_o [m/s]/1 -> Mux7/2, Mux5/2, Mux6/2
  Mux5/1 -> Delta P c7/1
  [Dh_c_o] -> Mux7/5
  csi_c4=csi_c6/1 -> Mux6/3
  Mux6/1 -> Delta P c9/1, Delta P c6/1
  Mux7/1 -> Delta P c8/1
  csi_c5/1 -> Mux5/3
  Delta P c7/1 -> Delta Pc7 [Pa]/1
  [E] -> Mux7/4
  Delta P c9/1 -> Delta Pc9 [Pa]/1
  Delta P c8/1 -> Delta Pc8 [Pa]/1
  Delta P c6/1 -> Delta Pc6 [Pa]/1
  reynolds_ar_o/1 -> Fator de atrito saída/1

== system simulink_validacao/Recuperdor de calor CWPS/Queda de Pressão Fluido Quente/Queda de pressão fluido quente na saida ==
  rho_h_o [kg/m3] : Inport
  um_h_o [m/s] : Inport  Port=2
  reynolds_gas_o : Inport  Port=3
  Delta P h5 : Fcn  Expr=u(3)*((u(1)*u(2)^2)/2)
  Delta P h6 : Fcn  Expr=u(3)*((u(4)+u(5))/(2*u(6)))*((u(1)*u(2)^2)/2)
  Delta P h7 : Fcn  Expr=u(3)*((u(1)*u(2)^2)/2)
  Fator de atrito fluido quente saida : Fcn  Expr=112/u(1)
  Mux1 : Mux  Inputs=6
  Mux2 : Mux  Inputs=3
  csi_h3=csi_h4 : Constant
  Delta Ph5 [Pa] : Outport
  Delta Ph6 [Pa] : Outport  Port=2
  Delta Ph7 [Pa] : Outport  Port=3
  wires:
  Mux2/1 -> Delta P h5/1, Delta P h7/1
  [A] -> Mux1/4
  csi_h3=csi_h4/1 -> Mux2/3
  Mux1/1 -> Delta P h6/1
  [Dh_h_o] -> Mux1/6
  Fator de atrito fluido quente saida/1 -> Mux1/3
  Delta P h5/1 -> Delta Ph5 [Pa]/1
  um_h_o [m/s]/1 -> Mux2/2, Mux1/2
  reynolds_gas_o/1 -> Fator de atrito fluido quente saida/1
  Delta P h6/1 -> Delta Ph6 [Pa]/1
  Delta P h7/1 -> Delta Ph7 [Pa]/1
  rho_h_o [kg/m3]/1 -> Mux2/1, Mux1/1
  [D] -> Mux1/5

== system simulink_validacao/Recuperdor de calor CWPS/Queda de Pressão Fluido Quente/Queda de pressão fluido quente adicional  ==
  rho_h_o [m/s] : Inport
  um_h_o [m/s] : Inport  Port=2
  um_h_i [m/s] : Inport  Port=3
  rho_h_i [kg/m3] : Inport  Port=4
  Delta P c10 : Fcn  Expr=(u(1)*u(2)^2)-(u(3)*u(4)^2)
  Mux9 : Mux
  Delta Pc10 [Pa] : Outport
  wires:
  Delta P c10/1 -> Delta Pc10 [Pa]/1
  Mux9/1 -> Delta P c10/1
  rho_h_i [kg/m3]/1 -> Mux9/1
  um_h_i [m/s]/1 -> Mux9/2
  rho_h_o [m/s]/1 -> Mux9/3
  um_h_o [m/s]/1 -> Mux9/4

== system simulink_validacao/Recuperdor de calor CWPS/Queda de Pressão Fluido Quente/Queda de pressão fluido quente na entrada ==
  reynolds_h_i : Inport
  rho_h_i [kg/m3] : Inport  Port=2
  um_h_i [m/s] : Inport  Port=3
  Delta P h1 : Fcn  Expr=u(3)*((u(1)*u(2)^2)/2)
  Delta P h2 : Fcn  Expr=u(3)*((u(4)+u(5))/(2*u(6)))*((u(1)*u(2)^2)/2)
  Delta P h3 : Fcn  Expr=u(3)*((u(1)*u(2)^2)/2)
  Fator de atrito fluido quente entrada : Fcn  Expr=112/u(1)
  Mux1 : Mux  Inputs=6
  Mux2 : Mux  Inputs=3
  csi_h1=csi_h2 : Constant  Value=0.5
  Delta Ph1 [Pa] : Outport
  Delta Ph2 [Pa] : Outport  Port=2
  Delta Ph3 [Pa] : Outport  Port=3
  wires:
  Mux2/1 -> Delta P h1/1, Delta P h3/1
  [A] -> Mux1/4
  csi_h1=csi_h2/1 -> Mux2/3
  Mux1/1 -> Delta P h2/1
  [Dh_h_i] -> Mux1/6
  Fator de atrito fluido quente entrada/1 -> Mux1/3
  Delta P h1/1 -> Delta Ph1 [Pa]/1
  um_h_i [m/s]/1 -> Mux1/2, Mux2/2
  reynolds_h_i/1 -> Fator de atrito fluido quente entrada/1
  Delta P h2/1 -> Delta Ph2 [Pa]/1
  Delta P h3/1 -> Delta Ph3 [Pa]/1
  rho_h_i [kg/m3]/1 -> Mux1/1, Mux2/1
  [D] -> Mux1/5

== system simulink_validacao/Recuperdor de calor CWPS/Queda de Pressão Fluido Quente/Queda de pressão fluido quente nos dutos CW ==
  rho_h_ch [kg/m3] : Inport
  um_h_ch [m/s] : Inport  Port=2
  reynolds_h_ch : Inport  Port=3
  Delta P h4 : Fcn  Expr=u(3)*(u(4)/u(5))*((u(1)*u(2)^2)/2)
  Display : Display
  Fator de atrito fluido quente canais : Fcn  Expr=u(2)*(112/u(1))
  Mux1 : Mux  Inputs=2
  Mux8 : Mux  Inputs=5
  kappa : Constant  Value=1.6
  Delta Ph4 [Pa] : Outport
  wires:
  Mux8/1 -> Delta P h4/1
  um_h_ch [m/s]/1 -> Mux8/2
  rho_h_ch [kg/m3]/1 -> Mux8/1
  [Dh_h_ch] -> Mux8/5
  Fator de atrito fluido quente canais/1 -> Mux8/3
  Delta P h4/1 -> Delta Ph4 [Pa]/1
  Mux1/1 -> Fator de atrito fluido quente canais/1
  reynolds_h_ch/1 -> Display/1, Mux1/1
  kappa/1 -> Mux1/2
  [B] -> Mux8/4
